simulink model "hw1"  (R2020a)
settings: Solver=VariableStepAuto  StartTime=0.0  StopTime=0.1  RelTol=1e-3
undefined symbols (not defined in the file): b, D2R, J, Ke, Kt, La, Ra, TL, Va
settings Model: Creator=helep  LastModifiedBy=JeongHun Hong
settings SFSimCC: CustomCodeUndefinedFunction=UseInterfaceOnly

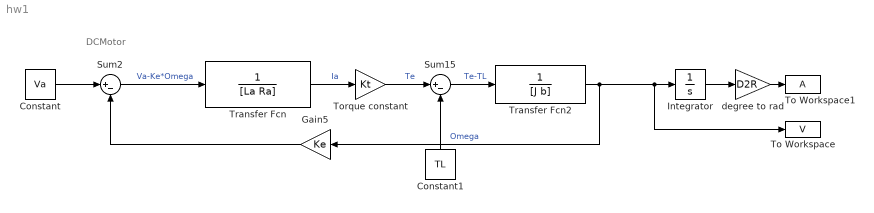
== system hw1 ==
  note: DCMotor
  Constant : Constant  Value=Va
  Constant1 : Constant  Value=TL
  Gain5 : Gain  Gain=Ke
  Integrator : Integrator
  Sum15 : Sum  Inputs=|+-
  Sum2 : Sum  Inputs=|+-
  To Workspace : ToWorkspace  VariableName=V  SaveFormat=Structure With Time  SampleTime=-1
  To Workspace1 : ToWorkspace  VariableName=A  SaveFormat=Structure With Time  SampleTime=-1
  Torque constant : Gain  Gain=Kt
  Transfer Fcn : TransferFcn  Denominator=[La Ra]
  Transfer Fcn2 : TransferFcn  Denominator=[J b]
  degree to rad : Gain  Gain=D2R
  wires:
  Integrator/1 -> degree to rad/1
  degree to rad/1 -> To Workspace1/1
  Transfer Fcn2/1 -> Gain5/1, Integrator/1, To Workspace/1  "Omega"
  Constant/1 -> Sum2/1
  Torque constant/1 -> Sum15/1  "Te"
  Sum15/1 -> Transfer Fcn2/1  "Te-TL"
  Constant1/1 -> Sum15/2
  Transfer Fcn/1 -> Torque constant/1  "Ia"
  Sum2/1 -> Transfer Fcn/1  "Va-Ke*Omega"
  Gain5/1 -> Sum2/2
